simulink model "Controller_BUG"  (R2019a)
settings: Solver=FixedStepDiscrete  StartTime=0.0  StopTime=10.0  FixedStep=0.005  RelTol=1e-3
libraries: simulink x4
settings Model: Creator=DELL  LastModifiedBy=DELL
settings DataIOCC: SaveFormat=Array
settings OptimizationCC: DefaultParameterBehavior=Inlined  EnhancedBackFolding=on  PassReuseOutputArgsAs=Individual arguments  OptimizeBlockOrder=speed  DifferentSizesBufferReuse=on  OptimizationCustomize=off
settings DebuggingCC: ParameterTunabilityLossMsg=error
settings SFSimCC: MATLABDynamicMemAlloc=off
settings RTWCC: SystemTargetFile=ert.tlc  GenCodeOnly=on  TemplateMakefile=ert_default_tmf  GenerateReport=on  IncludeHyperlinkInReport=on  LaunchReport=on  GenerateTraceInfo=on  GenerateTraceReport=on  GenerateTraceReportSl=on  GenerateTraceReportSf=on  GenerateTraceReportEml=on
settings CodeAppCC: ForceParamTrailComments=on  IgnoreCustomStorageClasses=off  OperatorAnnotations=on  SimulinkDataObjDesc=on  SFDataObjDesc=on  InsertBlockDesc=on
settings ERTTargetCC: TargetLangStandard=C99 (ISO)  GenerateSampleERTMain=on  InlinedParameterPlacement=NonHierarchical  ERTCustomFileTemplate=example_file_process.tlc

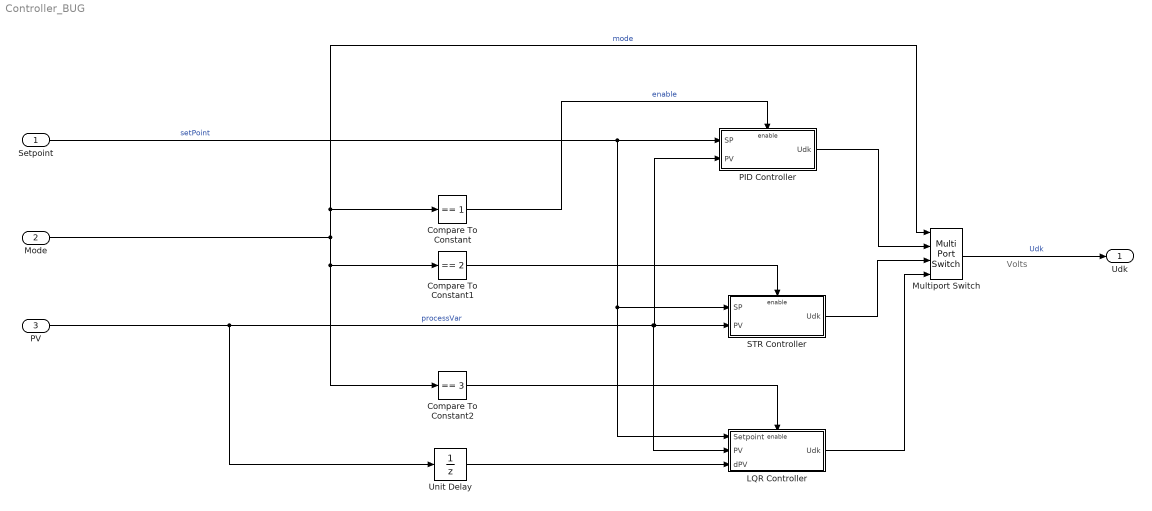
== system Controller_BUG ==
  note: Volts
  Setpoint : Inport
  Mode : Inport  Port=2
  PV : Inport  Port=3
  Compare To Constant : simulink/Logic and Bit Operations/Compare To Constant  relop===  const=1  OutDataTypeStr=boolean
  Compare To Constant1 : simulink/Logic and Bit Operations/Compare To Constant  relop===  const=2  OutDataTypeStr=boolean
  Compare To Constant2 : simulink/Logic and Bit Operations/Compare To Constant  relop===  const=3  OutDataTypeStr=boolean
  LQR Controller : Subsystem
  Multiport Switch : MultiPortSwitch
  PID Controller : Subsystem
  STR Controller : Subsystem
  Unit Delay : UnitDelay  SampleTime=-1  HasFrameUpgradeWarning=on
  Udk : Outport
  wires:
  Setpoint/1 -> LQR Controller/1(Setpoint), STR Controller/1(SP), PID Controller/1(SP)  "setPoint"
  PV/1 -> Unit Delay/1, LQR Controller/2(PV), STR Controller/2(PV), PID Controller/2(PV)  "processVar"
  Mode/1 -> Multiport Switch/1, Compare To Constant/1, Compare To Constant1/1, Compare To Constant2/1  "mode"
  Compare To Constant/1 -> PID Controller/Enable  "enable"
  Compare To Constant1/1 -> STR Controller/Enable
  Multiport Switch/1 -> Udk/1  "Udk"
  PID Controller/1(Udk) -> Multiport Switch/2
  STR Controller/1(Udk) -> Multiport Switch/3
  Compare To Constant2/1 -> LQR Controller/Enable
  LQR Controller/1(Udk) -> Multiport Switch/4
  Unit Delay/1 -> LQR Controller/3(dPV)

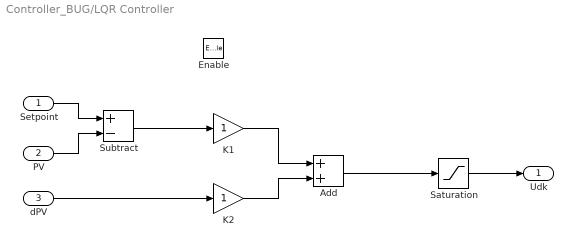
== system Controller_BUG/LQR Controller ==
  Setpoint : Inport
  PV : Inport  Port=2
  dPV : Inport  Port=3
  Enable : EnablePort
  Add : Sum
  K1 : Gain
  K2 : Gain
  Saturation : Saturate  UpperLimit=10  LowerLimit=-10
  Subtract : Sum  Inputs=+-
  Udk : Outport
  wires:
  Setpoint/1 -> Subtract/1
  PV/1 -> Subtract/2
  Saturation/1 -> Udk/1
  Add/1 -> Saturation/1
  K1/1 -> Add/1
  K2/1 -> Add/2
  Subtract/1 -> K1/1
  dPV/1 -> K2/1

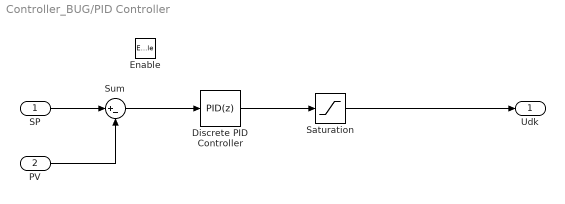
== system Controller_BUG/PID Controller ==
  SP : Inport
  PV : Inport  Port=2
  Enable : EnablePort
  Discrete PID Controller : simulink/Continuous/PID Controller  Controller=PID  Form=Parallel  TimeDomain=Discrete-time  SampleTime=-1  IntegratorMethod=Forward Euler  FilterMethod=Forward Euler  ControllerParametersSource=internal  P=1  I=1  D=0  UseFilter=on  N=100  TunerSelectOption=Transfer Function Based (PID Tuner App)  InitialConditionSource=internal  InitialConditionForIntegrator=0  InitialConditionForFilter=0  DifferentiatorICPrevScaledInput=0  ExternalReset=none  TrackingMode=off  Kt=1  LimitOutput=off  UpperSaturationLimit=inf  LowerSaturationLimit=-inf  LinearizeAsGain=off  AntiWindupMode=none  Kb=1  POutMin=[]  POutMax=[]  IOutMin=[]  IOutMax=[]  DOutMin=[]  DOutMax=[]  NOutMin=[]  NOutMax=[]  SumOutMin=[]  SumOutMax=[]  SaturationOutMin=[]  SaturationOutMax=[]  PParamMin=[]  PParamMax=[]  IParamMin=[]  IParamMax=[]  DParamMin=[]  DParamMax=[]  NParamMin=[]  NParamMax=[]  KbParamMin=[]  KbParamMax=[]  KtParamMin=[]  KtParamMax=[]  KbOutMin=[]  KbOutMax=[]  KtOutMin=[]  KtOutMax=[]  IntegratorOutMin=[]  IntegratorOutMax=[]  FilterOutMin=[]  FilterOutMax=[]  SumI1OutMin=[]  SumI1OutMax=[]  SumI2OutMin=[]  SumI2OutMax=[]  SumI3OutMin=[]  SumI3OutMax=[]  SumI4OutMin=[]  SumI4OutMax=[]  SumDOutMin=[]  SumDOutMax=[]  DifferentiatorOutMin=[]  DifferentiatorOutMax=[]  FilterDiffOutCoefMin=[]  FilterDiffOutCoefMax=[]  ReciprocalOutMin=[]  ReciprocalOutMax=[]  SumDenOutMin=[]  SumDenOutMax=[]  SumNumOutMin=[]  SumNumOutMax=[]  DivideOutMin=[]  DivideOutMax=[]  IntegratorContinuousStateAttributes=''  IntegratorStateMustResolveToSignalObject=off  IntegratorRTWStateStorageClass=Auto  FilterContinuousStateAttributes=''  FilterStateMustResolveToSignalObject=off  FilterRTWStateStorageClass=Auto  ParallelPVariant=InternalParameters  IdealPVariant=Disabled  IVariant=InternalParameters  DVariant=InternalParameters  IntegratorVariant=Discrete  SatVariant=Disabled  AWVariant=Passthrough  PCopyVariant=Disabled  TRVariant=Disabled  FdbkBlocksVariant=Forward  IdealPFdbkVariant=Disabled  SatFdbkVariant=Disabled  DerivativeFilterVariant=ForwardEulerFilter  NVariant=InternalParameters  NCopyVariant=Disabled  FilterICVariant=InternalICsFilter  IntegratorICVariant=InternalICs  ExternalResetVariant=Disabled  TRSumVariant=Passthrough  SumFdbkVariant=Disabled  SumVariant=Sum_PID
  Saturation : Saturate  UpperLimit=10  LowerLimit=-10
  Sum : Sum  Inputs=|+-
  Udk : Outport
  wires:
  SP/1 -> Sum/1
  PV/1 -> Sum/2
  Sum/1 -> Discrete PID Controller/1
  Discrete PID Controller/1 -> Saturation/1
  Saturation/1 -> Udk/1

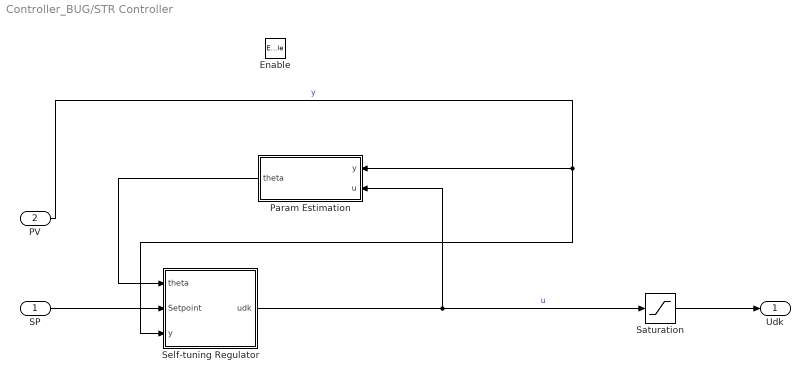
== system Controller_BUG/STR Controller ==
  SP : Inport
  PV : Inport  Port=2
  Enable : EnablePort
  Param Estimation : Subsystem
  Saturation : Saturate  UpperLimit=10  LowerLimit=-10
  "Self-tuning Regulator " : Subsystem
  Udk : Outport
  wires:
  PV/1 -> "Self-tuning Regulator "/3(y), Param Estimation/1("y ")  "y"
  "Self-tuning Regulator "/1(udk) -> Param Estimation/2(u), Saturation/1  "u"
  SP/1 -> "Self-tuning Regulator "/2(Setpoint)
  Param Estimation/1(theta) -> "Self-tuning Regulator "/1(theta)
  Saturation/1 -> Udk/1

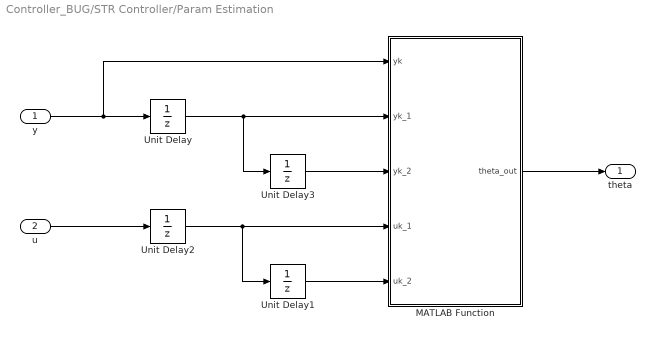
== system Controller_BUG/STR Controller/Param Estimation ==
  "y " : Inport  PortDimensions=1
  u : Inport  Port=2  PortDimensions=1
  MATLAB Function : MATLAB Function  TreatAsAtomicUnit=on
  Unit Delay{,1..3} (4 alike) : UnitDelay  SampleTime=-1  HasFrameUpgradeWarning=on
  theta : Outport  PortDimensions=4
  wires:
  "y "/1 -> MATLAB Function/1(yk), Unit Delay/1
  u/1 -> Unit Delay2/1
  MATLAB Function/1(theta_out) -> theta/1
  Unit Delay/1 -> Unit Delay3/1, MATLAB Function/2(yk_1)
  Unit Delay2/1 -> MATLAB Function/4(uk_1), Unit Delay1/1
  Unit Delay3/1 -> MATLAB Function/3(yk_2)
  Unit Delay1/1 -> MATLAB Function/5(uk_2)

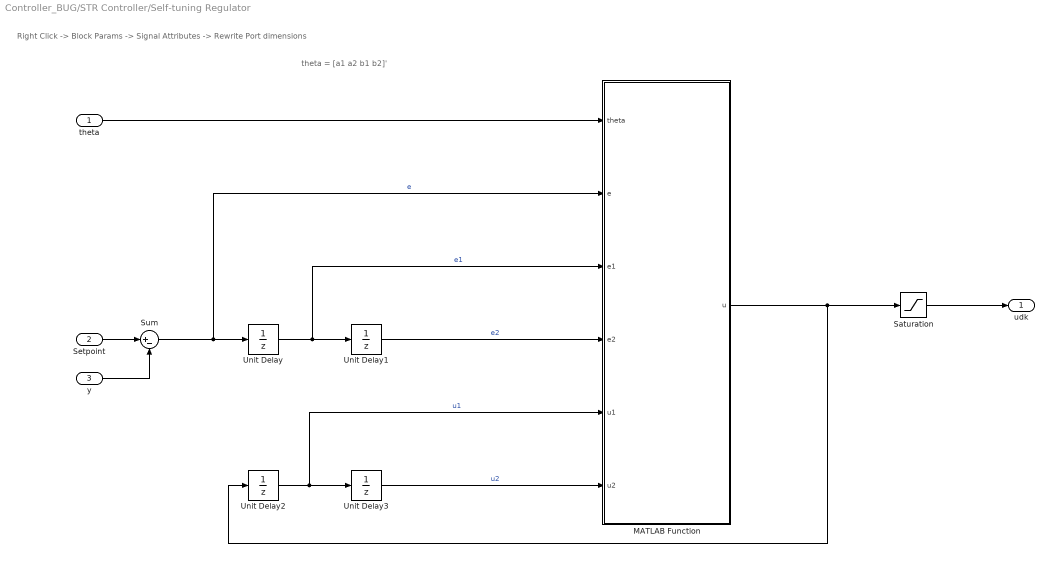
== system Controller_BUG/STR Controller/Self-tuning Regulator  ==
  note: Right Click -> Block Params -> Signal Attributes -> Rewrite Port dimensions
  note: theta = [a1 a2 b1 b2]'
  theta : Inport  PortDimensions=4
  Setpoint : Inport  Port=2  PortDimensions=1
  y : Inport  Port=3  PortDimensions=1
  MATLAB Function : MATLAB Function  TreatAsAtomicUnit=on
  Saturation : Saturate  UpperLimit=10  LowerLimit=-10
  Sum : Sum  Inputs=|+-
  Unit Delay{,1..3} (4 alike) : UnitDelay  SampleTime=-1  HasFrameUpgradeWarning=on
  udk : Outport  PortDimensions=1
  wires:
  Saturation/1 -> udk/1
  Setpoint/1 -> Sum/1
  y/1 -> Sum/2
  Sum/1 -> MATLAB Function/2(e), Unit Delay/1  "e"
  Unit Delay/1 -> MATLAB Function/3(e1), Unit Delay1/1  "e1"
  theta/1 -> MATLAB Function/1(theta)
  Unit Delay1/1 -> MATLAB Function/4(e2)  "e2"
  MATLAB Function/1(u) -> Saturation/1, Unit Delay2/1
  Unit Delay2/1 -> MATLAB Function/5(u1), Unit Delay3/1  "u1"
  Unit Delay3/1 -> MATLAB Function/6(u2)  "u2"

== matlab function Controller_BUG/STR Controller/Self-tuning Regulator /MATLAB Function ==
  data: theta input; u output; e input; e1 input; e2 input; u1 input; u2 input
function u = STR(theta,e,e1,e2,u1,u2)
T0 = 0.005;
xi = 0.99
wn = 20;
% Gan lai thong so de thuan tien viec tinh toan
a1 = theta(1);
a2 = theta(2);
b1 = theta(3);
b2 = theta(4);
% Tinh thong so bo dieu khien
if(xi<1)
d1 = -2*exp(-xi*wn*T0)*cos(wn*T0*sqrt(1-xi^2)); % xi<1
else
d1 = -2*exp(-xi*wn*T0)*cosh(wn*T0*sqrt(xi^2-1)); % xi>1
end
d2 = exp(-2*xi*wn*T0);
r1 = (b1+b2)*(a1*b1*b2-a2*b1*b1-b2*b2);
s1 = a2*((b1+b2)*(a1*b2-a2*b1)+b2*(b1*d2-b2*d1-b2));
q2 = s1/r1;
gamma = q2*b2/a2;
q1 = a2/b2-q2*(b1/b2-a1/a2+1);
q0 = (d1+1-a1-gamma)/b1;
% Luat dieu khien
u = q0*e + q1*e1 + q2*e2 + (1-gamma)*u1+ gamma*u2;

== matlab function Controller_BUG/STR Controller/Param Estimation/MATLAB Function ==
  data: yk input; yk_1 input; yk_2 input; uk_1 input; theta_out output; uk_2 input
function theta_out = fcn(yk,yk_1,yk_2,uk_1,uk_2)
persistent theta P

if (isempty(theta))
    theta = rand(4,1);
    P = 10*eye(4);
end

lambda = 0.995;

phi = [-yk_1;-yk_2;uk_1;uk_2];

Lk = P*phi/(lambda + phi'*P*phi);
P = 1/lambda*(P-Lk*phi'*P);
ek = yk - phi'*theta;
theta = theta + Lk*ek;

theta_out = theta;
end
